simulink model "MPC_backend"  (R2026a)
settings: Solver=VariableStepAuto
model workspace (MAT data in the model file):
  kappa_ref = 1
  mpc_ref = 1
libraries: mpclib x1
settings Model: Creator=rayyu  LastModifiedBy=rayyu

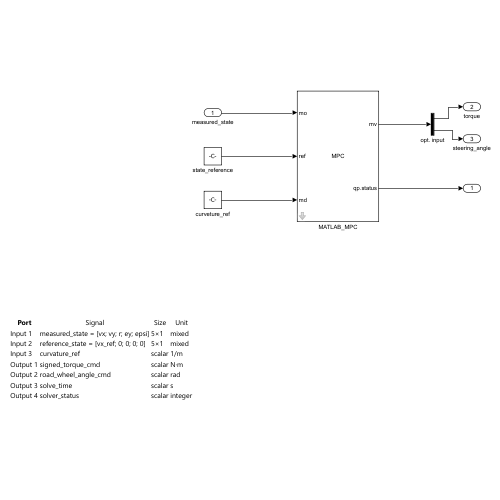
[thumbnail: Simulink's stored preview of the top-level diagram]
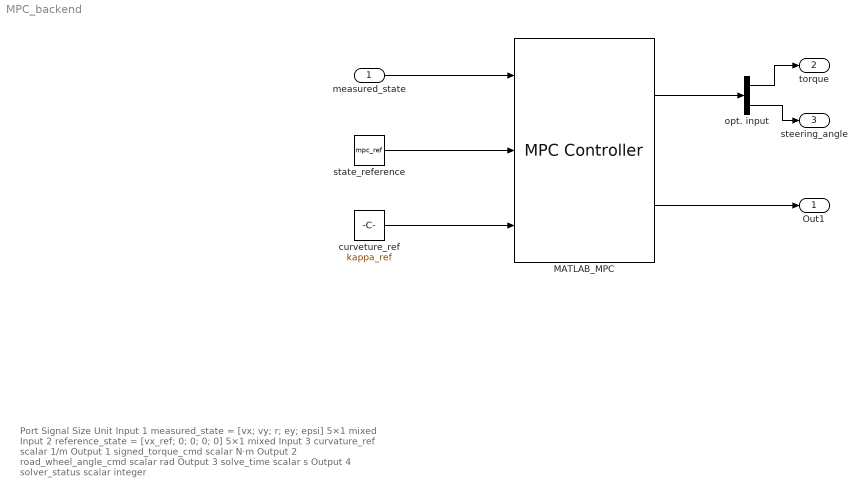
== system MPC_backend ==
  note: Port
      | Signal
      | Size
      | Unit
      |
      | Input 1
      | measured_state = [vx; vy; r; ey; epsi]
      | 5×1
      | mixed
      |
      | Input 2
      | reference_state = [vx_ref; 0; 0; 0; 0]
      | 5×1
      | mixed
      |
      | Input 3
      | curvature_ref
      | scalar
      | 1/m
      |
      | Output 1
      | signed_torque_cmd
      | scalar
      | N·m
      |
      | Output 2
      | road_wheel_angle_cmd
      | scalar
      | rad
      |
      | Output 3
      | solve_time
      | scalar
      | s
      |
      | Output 4
      | solver_status
      | scalar
      | integer
  measured_state : Inport
  MATLAB_MPC : mpclib/MPC Controller  SCDEnableBlockLinearizationSpecification=on  mpcobj=mpc_baseline  is_multiple=0  enable_value=0  return_u0=off  updateMPCinCallerWorkspace=on  md_inport=on  mv_inport=off  uref_inport=off  return_cost=off  return_mvseq=off  return_qpstatus=on  return_xseq=off  return_state=off  return_ovseq=off  state_inport=off  umin_inport=off  umax_inport=off  ymin_inport=off  ymax_inport=off  cc_inport=off  ywt_inport=off  uwt_inport=off  duwt_inport=off  rhoeps_inport=off  pm_inport=off  MaximumP=10  HorizonChoice=FixedHorizon  n_ts=1  n_p=10  n_mv=1  n_md=1  n_ud=0  n_mo=1  n_uo=0  BlockDataType=double  SampleTimeInherited=off  switch_inport=off
  curveture_ref : Constant  Value=kappa_ref
  opt. input : Demux  Outputs=2
  state_reference : Constant  Value=mpc_ref
  Out1 : Outport
  torque : Outport  Port=2
  steering_angle : Outport  Port=3
  wires:
  MATLAB_MPC/1 -> opt. input/1
  MATLAB_MPC/2 -> Out1/1
  state_reference/1 -> MATLAB_MPC/2
  measured_state/1 -> MATLAB_MPC/1
  curveture_ref/1 -> MATLAB_MPC/3
  opt. input/1 -> torque/1
  opt. input/2 -> steering_angle/1
